simulink model "simulation"  (Simulink 8.8)
settings: Solver=ode45  StartTime=0.0  StopTime=max(t_simulink)  RelTol=1e-3  EnableMultiTasking=on
values from neighbouring files (symbols this model uses):
  fe_simulink = 50000    [TP.m]
libraries: librairie x7
settings Model: Creator=sylar  LastModifiedBy=3520807
settings OptimizationCC: ExpressionDepthLimit=2147483647
settings DebuggingCC: SolverPrmCheckMsg=warning  AllowSymbolicDim=off

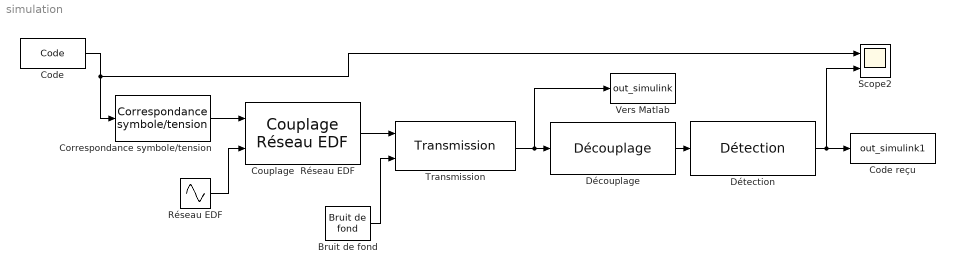
== system simulation ==
  Bruit de fond : librairie/Bruit de fond  RSB=-2
  Code : librairie/Code  T_symbole=Tsymbole_simulink
  Code reçu : ToWorkspace  VariableName=out_simulink1  SampleTime=-1
  Correspondance symbole/tension : librairie/Correspondance symbole//tension  A_symbole=Asymbole_simulink
  Couplage  Réseau EDF : librairie/Couplage  Réseau EDF  fp=10000
  Découplage : librairie/Découplage  TOTO=0
      link override Sine Wave: Frequency=2*pi*fp
  Détection : librairie/Détection  seuil=0
  Réseau EDF : Sin  Amplitude=sqrt(2)*240  Frequency=2*pi*50  SampleTime=0
  Scope2 : Scope  NumInputPorts=2
  Transmission : librairie/Transmission  TOTO=[]
  Vers Matlab : ToWorkspace  VariableName=out_simulink  SampleTime=1/fe_simulink
  wires:
  Code/1 -> Scope2/1, Correspondance symbole/tension/1
  Correspondance symbole/tension/1 -> Couplage  Réseau EDF/1
  Bruit de fond/1 -> Transmission/2
  Découplage/1 -> Détection/1
  Détection/1 -> Code reçu/1, Scope2/2
  Couplage  Réseau EDF/1 -> Transmission/1
  Réseau EDF/1 -> Couplage  Réseau EDF/2
  Transmission/1 -> Vers Matlab/1, Découplage/1
